simulink model "MEEN432_Project4_Model_V2"  (R2024b)
settings: Solver=VariableStepAuto  StartTime=0.0  StopTime=3600  RelTol=1e-3
values from neighbouring files (symbols this model uses):
  mph2mps = 1600/3600    (= 0.444444444444)    [Project4_init.m]
  x_track = zeros(size(s))    [Project4_track.m]
  y_track = zeros(size(s))    [Project4_track.m]
undefined symbols (not defined in the file or in its folder): datBat, datCar, datMotor
libraries: slpidlib x1
settings Model: Creator=flare  LastModifiedBy=jpalm
settings RTWCC: GPUComputeCapability=3.5

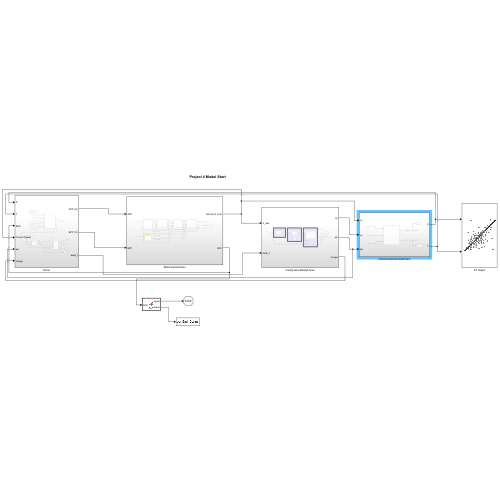
[thumbnail: Simulink's stored preview of the top-level diagram]
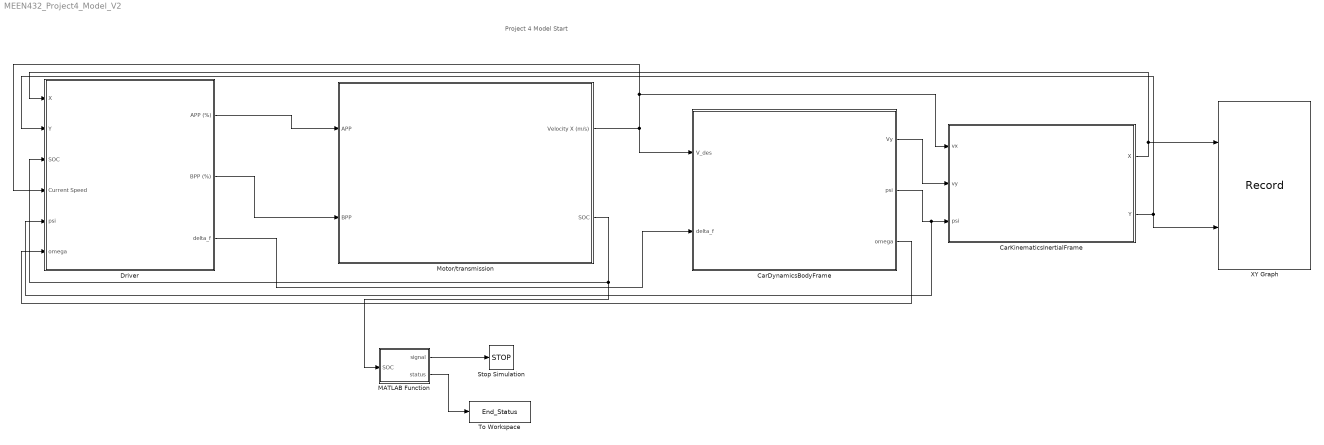
== system MEEN432_Project4_Model_V2 ==
  note: Project 4 Model Start
  CarDynamicsBodyFrame : Subsystem
  CarKinematicsInertialFrame : Subsystem
  Driver : Subsystem
  MATLAB Function : MATLAB Function  TreatAsAtomicUnit=on
  Motor/transmission : Subsystem
  Stop Simulation : Stop
  To Workspace : ToWorkspace  VariableName=End_Status  SaveFormat=Timeseries  SampleTime=-1
  XY Graph : Record  FileSettingsInternal="{\"entries\":[{\"content\":{\"excelSettings\":{\"content\":{},\"type\":\"Streamout.ExcelSettings\"}},\"type\":\"Streamout.FileSettingStorage\",\"uuid\":\"\"}],\"packageUris\":[\"http:\\/\\/schema.mathworks.com\\/mf0\\/streamout_blocks\\/R2020a\"],\"version\":\"1.0\"}"  Layout=[1 1]  SignalsInternal="{\"entries\":[{\"content\":{\"signals\":[{\"content\":{\"blockPath\":[],\"dimensions\":[1],\"domain\":\"\",\"lineColor\":\"#4dbeee\",\"plots\":[ 1 ],\"port\":1,\"sid\":[\"\"],\"signalID\":1,\"signalName\":\"CarKinematicsInertialFrame:1\"},\"type\":\"RecordBlkView.Signal\",\"uuid\":\"\"},{\"content\":{\"blockPath\":[],\"dimensions\":[1],\"domain\":\"\",\"lineColor\":\"#a2142f\",\"plots\":[ 1 ],\"port\":2,\"sid\":[\"\"],\"signalID\":2,\"signalName\":\"CarKinematicsInertialFrame:2\"},\"type\":\"RecordBlkView.Signal\",\"uuid\":\"\"}]},\"type\":\"RecordBlkView.InputSignals\",\"uuid\":\"\"}],\"packageUris\":[\"http:\\/\\/schema.mathworks.com\\/mf0\\/streamout_blocks\\/R2020a\"],\"version\":\"1.0\"}"  VisualizationBindings="{\"xyplotplugin\":{\"info\":[{\"series\":[{\"bindingParametersList\":[{\"parameter\":\"X-Axis\",\"signalID\":1,\"signalName\":\"CarKinematicsInertialFrame:1\"},{\"parameter\":\"Y-Axis\",\"signalID\":2,\"signalName\":\"CarKinematicsInertialFrame:2\"}],\"seriesID\":0}],\"subplotID\":1}]}}"  CompatibilityTag=XY
  wires:
  CarKinematicsInertialFrame/1(X) -> XY Graph/1, Driver/1(X)
  CarKinematicsInertialFrame/2(Y) -> XY Graph/2, Driver/2(Y)
  Driver/1(APP (%)) -> Motor/transmission/1(APP)
  Driver/2(BPP (%)) -> Motor/transmission/2(BPP)
  Driver/3(delta_f) -> CarDynamicsBodyFrame/2(delta_f)
  Motor/transmission/1(Velocity X (m/s)) -> Driver/4(Current Speed), CarKinematicsInertialFrame/1(vx), CarDynamicsBodyFrame/1(V_des)
  CarDynamicsBodyFrame/1(Vy) -> CarKinematicsInertialFrame/2(vy)
  CarDynamicsBodyFrame/2(psi) -> Driver/5(psi), CarKinematicsInertialFrame/3(psi)
  CarDynamicsBodyFrame/3(omega) -> Driver/6(omega)
  Motor/transmission/2(SOC) -> MATLAB Function/1(SOC), Driver/3(SOC)
  MATLAB Function/1(signal) -> Stop Simulation/1
  MATLAB Function/2(status) -> To Workspace/1

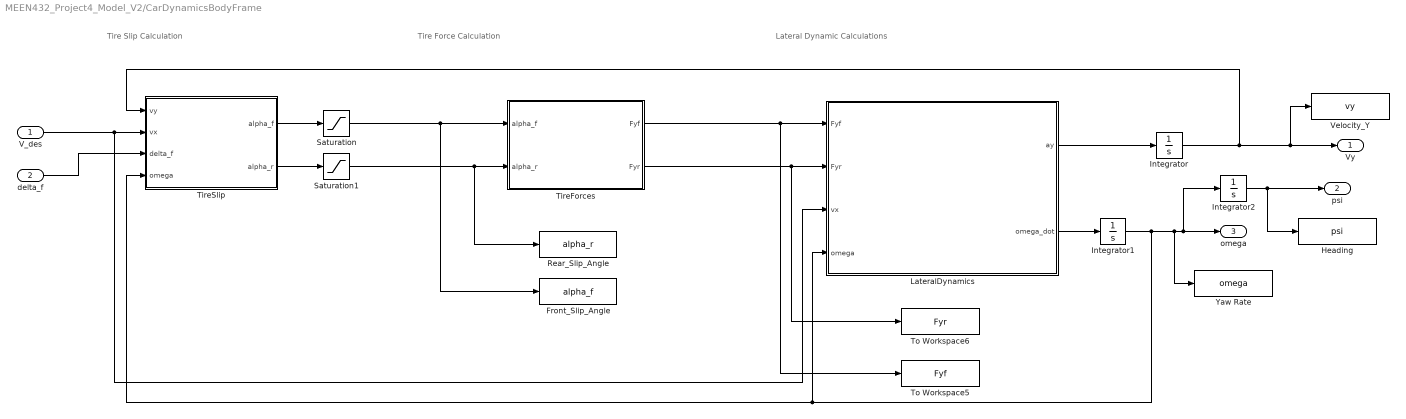
== system MEEN432_Project4_Model_V2/CarDynamicsBodyFrame ==
  note: Lateral Dynamic Calculations
  note: Tire Force Calculation
  note: Tire Slip Calculation
  V_des : Inport
  delta_f : Inport  Port=2
  Front_Slip_Angle : ToWorkspace  VariableName=alpha_f  SaveFormat=Timeseries  SampleTime=-1
  Heading : ToWorkspace  VariableName=psi  SaveFormat=Timeseries  SampleTime=-1
  Integrator : Integrator  InitialCondition=datCar.init.vy0
  Integrator1 : Integrator  InitialCondition=datCar.init.omega0
  Integrator2 : Integrator  InitialCondition=datCar.init.psi0
  LateralDynamics : MATLAB Function  TreatAsAtomicUnit=on  mask{obj=datCar}
      mask prompts: obj "obj structure"
  Rear_Slip_Angle : ToWorkspace  VariableName=alpha_r  SaveFormat=Timeseries  SampleTime=-1
  Saturation : Saturate  UpperLimit=datCar.maxAlpha  LowerLimit=-datCar.maxAlpha
  Saturation1 : Saturate  UpperLimit=datCar.maxAlpha  LowerLimit=-datCar.maxAlpha
  TireForces : MATLAB Function  TreatAsAtomicUnit=on  mask{obj=datCar}
      mask prompts: obj "obj structure"
  TireSlip : MATLAB Function  TreatAsAtomicUnit=on  mask{obj=datCar}
      mask prompts: obj "obj structure"
  To Workspace5 : ToWorkspace  VariableName=Fyf  SaveFormat=Timeseries  SampleTime=-1
  To Workspace6 : ToWorkspace  VariableName=Fyr  SaveFormat=Timeseries  SampleTime=-1
  Velocity_Y : ToWorkspace  VariableName=vy  SaveFormat=Timeseries  SampleTime=-1
  Yaw Rate : ToWorkspace  VariableName=omega  SaveFormat=Timeseries  SampleTime=-1
  Vy : Outport
  psi : Outport  Port=2
  omega : Outport  Port=3
  wires:
  delta_f/1 -> TireSlip/3(delta_f)
  V_des/1 -> TireSlip/2(vx), LateralDynamics/3(vx)
  Integrator2/1 -> Heading/1, psi/1
  Integrator1/1 -> Integrator2/1, omega/1, Yaw Rate/1, LateralDynamics/4(omega), TireSlip/4(omega)
  Saturation1/1 -> TireForces/2(alpha_r), Rear_Slip_Angle/1
  Saturation/1 -> TireForces/1(alpha_f), Front_Slip_Angle/1
  TireForces/1(Fyf) -> LateralDynamics/1(Fyf), To Workspace5/1
  LateralDynamics/1(ay) -> Integrator/1
  TireSlip/2(alpha_r) -> Saturation1/1
  TireSlip/1(alpha_f) -> Saturation/1
  TireForces/2(Fyr) -> LateralDynamics/2(Fyr), To Workspace6/1
  Integrator/1 -> Vy/1, Velocity_Y/1, TireSlip/1(vy)
  LateralDynamics/2(omega_dot) -> Integrator1/1

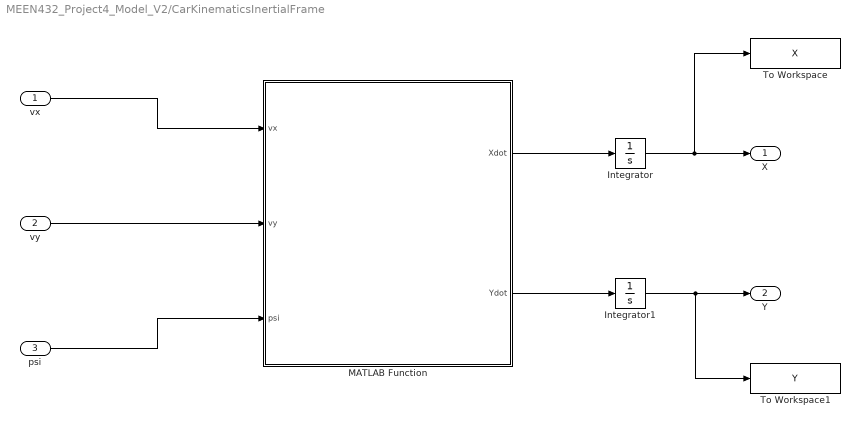
== system MEEN432_Project4_Model_V2/CarKinematicsInertialFrame ==
  vx : Inport
  vy : Inport  Port=2
  psi : Inport  Port=3
  Integrator : Integrator  InitialCondition=datCar.init.X0
  Integrator1 : Integrator  InitialCondition=datCar.init.Y0
  MATLAB Function : MATLAB Function  TreatAsAtomicUnit=on
  To Workspace : ToWorkspace  VariableName=X  SaveFormat=Timeseries  SampleTime=-1
  To Workspace1 : ToWorkspace  VariableName=Y  SaveFormat=Timeseries  SampleTime=-1
  X : Outport
  Y : Outport  Port=2
  wires:
  MATLAB Function/2(Ydot) -> Integrator1/1
  psi/1 -> MATLAB Function/3(psi)
  vx/1 -> MATLAB Function/1(vx)
  Integrator/1 -> To Workspace/1, X/1
  MATLAB Function/1(Xdot) -> Integrator/1
  Integrator1/1 -> To Workspace1/1, Y/1
  vy/1 -> MATLAB Function/2(vy)

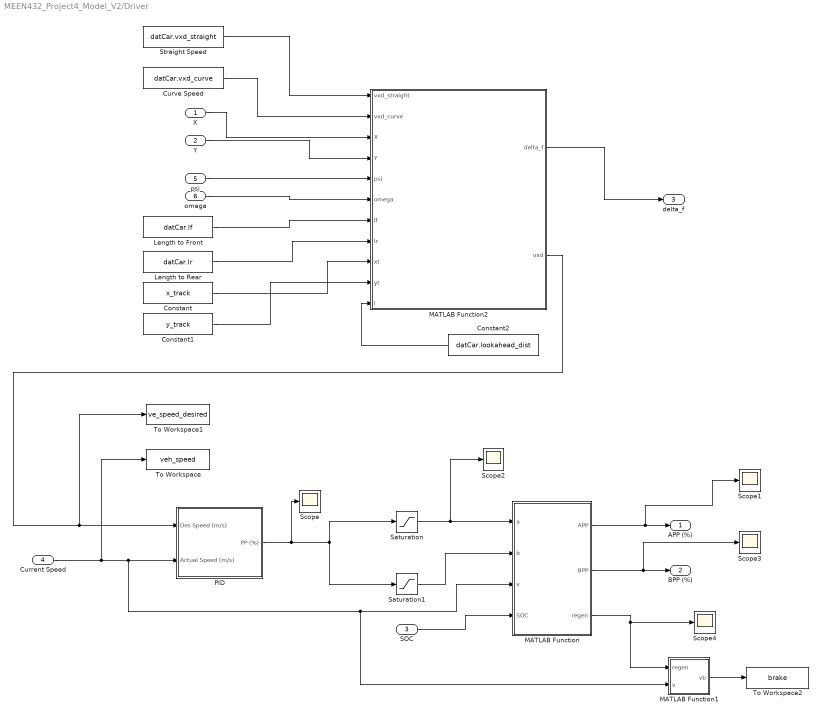
== system MEEN432_Project4_Model_V2/Driver ==
  X : Inport
  Y : Inport  Port=2
  SOC : Inport  Port=3
  Current Speed : Inport  Port=4
  psi : Inport  Port=5
  omega : Inport  Port=6
  Constant : Constant  Value=x_track  VectorParams1D=off
  Constant1 : Constant  Value=y_track  VectorParams1D=off
  Constant2 : Constant  Value=datCar.lookahead_dist
  Curve Speed : Constant  Value=datCar.vxd_curve
  Length to Front : Constant  Value=datCar.lf
  Length to Rear : Constant  Value=datCar.lr
  MATLAB Function : MATLAB Function  TreatAsAtomicUnit=on
  MATLAB Function1 : MATLAB Function  TreatAsAtomicUnit=on
  MATLAB Function2 : MATLAB Function  TreatAsAtomicUnit=on
  PID : Subsystem
  Saturation : Saturate  UpperLimit=1  LowerLimit=0
  Saturation1 : Saturate  UpperLimit=0  LowerLimit=-1
  Scope{,1..4} (5 alike) : Scope
  Straight Speed : Constant  Value=datCar.vxd_straight
  To Workspace : ToWorkspace  VariableName=veh_speed  SaveFormat=Timeseries  SampleTime=-1
  To Workspace1 : ToWorkspace  VariableName=ve_speed_desired  SaveFormat=Timeseries  SampleTime=-1
  To Workspace2 : ToWorkspace  VariableName=brake  SaveFormat=Timeseries  SampleTime=-1
  APP (%) : Outport
  BPP (%) : Outport  Port=2
  delta_f : Outport  Port=3
  wires:
  Current Speed/1 -> To Workspace/1, MATLAB Function1/2(v), MATLAB Function/3(v), PID/2(Actual Speed (m/s))
  MATLAB Function/1(APP) -> APP (%)/1, Scope1/1
  SOC/1 -> MATLAB Function/4(SOC)
  Saturation/1 -> Scope2/1, MATLAB Function/1(a)
  MATLAB Function/3(regen) -> MATLAB Function1/1(regen), Scope4/1
  MATLAB Function/2(BPP) -> BPP (%)/1, Scope3/1
  Saturation1/1 -> MATLAB Function/2(b)
  PID/1(PP (%)) -> Scope/1, Saturation1/1, Saturation/1
  MATLAB Function1/1(vb) -> To Workspace2/1
  Constant2/1 -> MATLAB Function2/11(l)
  Constant/1 -> MATLAB Function2/9(xt)
  Length to Rear/1 -> MATLAB Function2/8(lr)
  MATLAB Function2/1(delta_f) -> delta_f/1
  Constant1/1 -> MATLAB Function2/10(yt)
  X/1 -> MATLAB Function2/3(X)
  Y/1 -> MATLAB Function2/4(Y)
  Length to Front/1 -> MATLAB Function2/7(lf)
  Straight Speed/1 -> MATLAB Function2/1(vxd_straight)
  omega/1 -> MATLAB Function2/6(omega)
  psi/1 -> MATLAB Function2/5(psi)
  MATLAB Function2/2(vxd) -> To Workspace1/1, PID/1(Des Speed (m/s))
  Curve Speed/1 -> MATLAB Function2/2(vxd_curve)

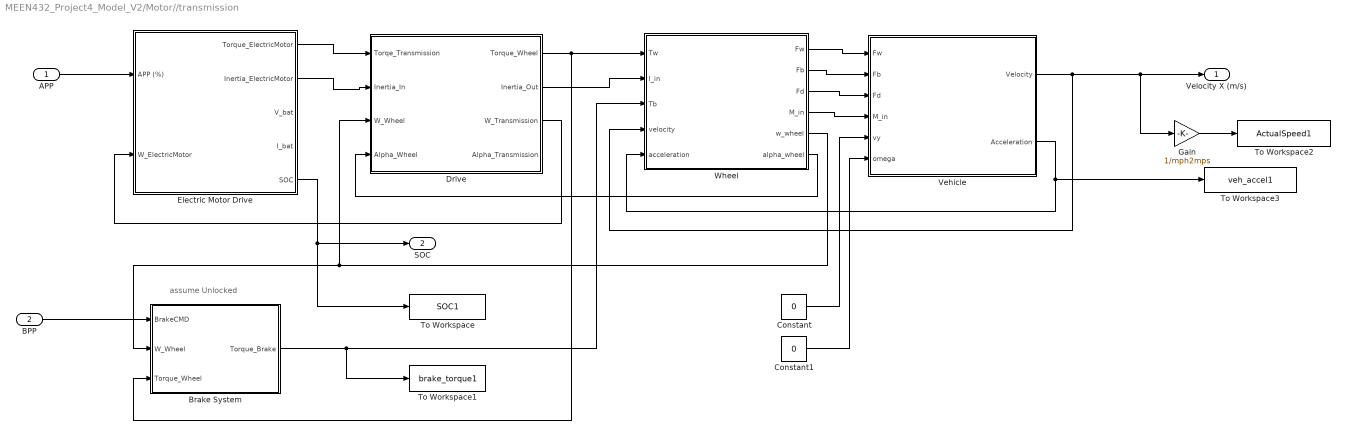
== system MEEN432_Project4_Model_V2/Motor//transmission ==
  note: assume Unlocked
  APP : Inport
  BPP : Inport  Port=2
  Brake System : Subsystem
  Constant : Constant  Value=0
  Constant1 : Constant  Value=0
  Drive : Subsystem
  Electric Motor Drive : Subsystem
  Gain : Gain  Gain=1/mph2mps
  To Workspace : ToWorkspace  VariableName=SOC1  SaveFormat=Timeseries  SampleTime=-1
  To Workspace1 : ToWorkspace  VariableName=brake_torque1  SaveFormat=Timeseries  SampleTime=-1
  To Workspace2 : ToWorkspace  VariableName=ActualSpeed1  SaveFormat=Timeseries  SampleTime=-1
  To Workspace3 : ToWorkspace  VariableName=veh_accel1  SaveFormat=Timeseries  SampleTime=-1
  Vehicle : Subsystem
  Wheel : Subsystem
  Velocity X (m/s) : Outport
  SOC : Outport  Port=2
  wires:
  Drive/3(W_Transmission) -> Electric Motor Drive/2(W_ElectricMotor)
  Drive/1(Torque_Wheel) -> Brake System/3(Torque_Wheel), Wheel/1(Tw)
  Brake System/1(Torque_Brake) -> To Workspace1/1, Wheel/3(Tb)
  Drive/2(Inertia_Out) -> Wheel/2(I_in)
  Wheel/1(Fw) -> Vehicle/1(Fw)
  Wheel/3(Fd) -> Vehicle/3(Fd)
  APP/1 -> Electric Motor Drive/1(APP (%))
  Vehicle/1(Velocity) -> Wheel/4(velocity), Gain/1, Velocity X (m/s)/1
  Wheel/2(Fb) -> Vehicle/2(Fb)
  Constant/1 -> Vehicle/5(vy)
  BPP/1 -> Brake System/1(BrakeCMD)
  Vehicle/2(Acceleration) -> To Workspace3/1, Wheel/5(acceleration)
  Electric Motor Drive/2(Inertia_ElectricMotor) -> Drive/2(Inertia_In)
  Gain/1 -> To Workspace2/1
  Constant1/1 -> Vehicle/6(omega)
  Electric Motor Drive/1(Torque_ElectricMotor) -> Drive/1(Torqe_Transmission)
  Wheel/6(alpha_wheel) -> Drive/4(Alpha_Wheel)
  Wheel/4(M_in) -> Vehicle/4(M_in)
  Electric Motor Drive/5(SOC) -> To Workspace/1, SOC/1
  Wheel/5(w_wheel) -> Drive/3(W_Wheel), Brake System/2(W_Wheel)

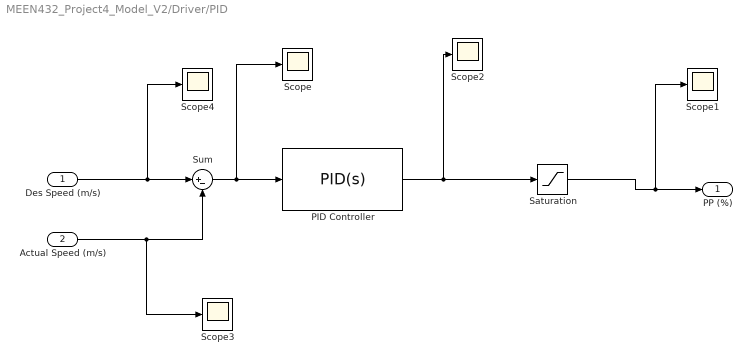
== system MEEN432_Project4_Model_V2/Driver/PID ==
  Des Speed (m/s) : Inport
  Actual Speed (m/s) : Inport  Port=2
  PID Controller : slpidlib/PID Controller  Controller=PID  Form=Parallel  TimeDomain=Continuous-time  UseExternalTs=off  SampleTime=-1  IntegratorMethod=Forward Euler  FilterMethod=Forward Euler  ControllerParametersSource=internal  P=1  I=1  UseKiTs=off  D=0  UseExternalDerivativeSource=off  N=100  UseFilter=on  TunerSelectOption=Transfer Function Based (PID Tuner App)  InitialConditionSource=internal  InitialConditionForIntegrator=0  InitialConditionForFilter=0  DifferentiatorICPrevScaledInput=0  ExternalReset=none  TrackingMode=off  Kt=1  LimitOutput=off  SatLimitsSource=internal  UpperSaturationLimit=inf  LowerSaturationLimit=-inf  LinearizeAsGain=on  AntiWindupMode=none  Kb=1  LimitIntegrator=off  UpperIntegratorSaturationLimit=inf  LowerIntegratorSaturationLimit=-inf  POutMin=[]  POutMax=[]  IOutMin=[]  IOutMax=[]  DOutMin=[]  DOutMax=[]  NOutMin=[]  NOutMax=[]  SumOutMin=[]  SumOutMax=[]  SaturationOutMin=[]  SaturationOutMax=[]  PParamMin=[]  PParamMax=[]  IParamMin=[]  IParamMax=[]  DParamMin=[]  DParamMax=[]  NParamMin=[]  NParamMax=[]  KbParamMin=[]  KbParamMax=[]  KtParamMin=[]  KtParamMax=[]  KbOutMin=[]  KbOutMax=[]  KtOutMin=[]  KtOutMax=[]  IntegratorOutMin=[]  IntegratorOutMax=[]  FilterOutMin=[]  FilterOutMax=[]  SumI1OutMin=[]  SumI1OutMax=[]  SumI2OutMin=[]  SumI2OutMax=[]  SumI3OutMin=[]  SumI3OutMax=[]  SumI4OutMin=[]  SumI4OutMax=[]  SumDOutMin=[]  SumDOutMax=[]  DifferentiatorOutMin=[]  DifferentiatorOutMax=[]  FilterDiffOutCoefMin=[]  FilterDiffOutCoefMax=[]  ReciprocalOutMin=[]  ReciprocalOutMax=[]  SumDenOutMin=[]  SumDenOutMax=[]  SumNumOutMin=[]  SumNumOutMax=[]  DivideOutMin=[]  DivideOutMax=[]  UdiffTsProdOutMin=[]  UdiffTsProdOutMax=[]  NTsProdOutMin=[]  NTsProdOutMax=[]  UintegralTsProdOutMin=[]  UintegralTsProdOutMax=[]  UngainTsProdOutMin=[]  UngainTsProdOutMax=[]  ClampingZeroOutDataTypeStr=Inherit: Inherit via back propagation  ClampingZeroOutMin=[]  ClampingZeroOutMax=[]  FilterDenConstantOutDataTypeStr=Inherit: Inherit via back propagation  FilterDenConstantOutMin=[]  FilterDenConstantOutMax=[]  PCopyOutDataTypeStr=Inherit: Inherit via back propagation  PCopyOutMin=[]  PCopyOutMax=[]  NCopyOutDataTypeStr=Inherit: Inherit via back propagation  NCopyOutMin=[]  NCopyOutMax=[]  IntegratorContinuousStateAttributes=''  IntegratorStateMustResolveToSignalObject=off  IntegratorRTWStateStorageClass=Auto  FilterContinuousStateAttributes=''  FilterStateMustResolveToSignalObject=off  FilterRTWStateStorageClass=Auto  ParallelPVariant=InternalParameters  IdealPVariant=Disabled  IVariant=InternalParameters  DVariant=InternalParameters  IntegratorVariant=Continuous  SatVariant=Disabled  AWVariant=Passthrough  PCopyVariant=Disabled  TRVariant=Disabled  FdbkBlocksVariant=Forward  IdealPFdbkVariant=Disabled  SatFdbkVariant=Disabled  DerivativeFilterVariant=ContFilter  NVariant=InternalParameters  NCopyVariant=Disabled  FilterICVariant=InternalICsFilter  IntegratorICVariant=InternalICs  ExternalResetVariant=Disabled  TRSumVariant=Passthrough  SumFdbkVariant=Disabled  SumVariant=Sum_PID  TsampFilterVariant=InternalTs  TsampNgainVariant=Passthrough  TsampIntegralVariant=Disabled_SignalSpec  ExternalSaturationOutDataTypeStr=Inherit: Same as second input  DerivativeSourceVariant=ErrorSignal  PreIntVariant=InternalPreInt
  Saturation : Saturate  UpperLimit=1  LowerLimit=-1
  Scope{,1..4} (5 alike) : Scope
  Sum : Sum  Inputs=|+-
  PP (%) : Outport
  wires:
  Sum/1 -> Scope/1, PID Controller/1
  PID Controller/1 -> Saturation/1, Scope2/1
  Des Speed (m/s)/1 -> Scope4/1, Sum/1
  Actual Speed (m/s)/1 -> Scope3/1, Sum/2
  Saturation/1 -> Scope1/1, PP (%)/1

== system MEEN432_Project4_Model_V2/Motor//transmission/Brake System ==
  BrakeCMD : Inport
  W_Wheel : Inport  Port=2
  Torque_Wheel : Inport  Port=3
  Constant : Constant  Value=datCar.maxBrakeTorque
  Constant1 : Constant  Value=datCar.brakeGeometricDesign
  Constant2 : Constant  Value=datCar.brakeFriction
  MATLAB Function : MATLAB Function  TreatAsAtomicUnit=on
  Scope : Scope
  Torque_Brake : Outport
  wires:
  BrakeCMD/1 -> MATLAB Function/1(alpha_b)
  W_Wheel/1 -> MATLAB Function/5(omega_w)
  MATLAB Function/1(tau_b) -> Scope/1, Torque_Brake/1
  Constant/1 -> MATLAB Function/3(N_b_max)
  Constant1/1 -> MATLAB Function/4(g_b)
  Constant2/1 -> MATLAB Function/2(mu_b)

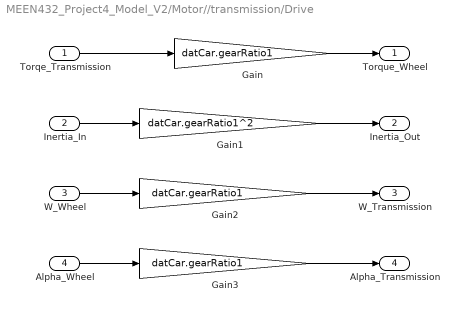
== system MEEN432_Project4_Model_V2/Motor//transmission/Drive ==
  Torqe_Transmission : Inport
  Inertia_In : Inport  Port=2
  W_Wheel : Inport  Port=3
  Alpha_Wheel : Inport  Port=4
  Gain : Gain  Gain=datCar.gearRatio1
  Gain1 : Gain  Gain=datCar.gearRatio1^2
  Gain2 : Gain  Gain=datCar.gearRatio1
  Gain3 : Gain  Gain=datCar.gearRatio1
  Torque_Wheel : Outport
  Inertia_Out : Outport  Port=2
  W_Transmission : Outport  Port=3
  Alpha_Transmission : Outport  Port=4
  wires:
  Torqe_Transmission/1 -> Gain/1
  Inertia_In/1 -> Gain1/1
  W_Wheel/1 -> Gain2/1
  Alpha_Wheel/1 -> Gain3/1
  Gain3/1 -> Alpha_Transmission/1
  Gain2/1 -> W_Transmission/1
  Gain1/1 -> Inertia_Out/1
  Gain/1 -> Torque_Wheel/1

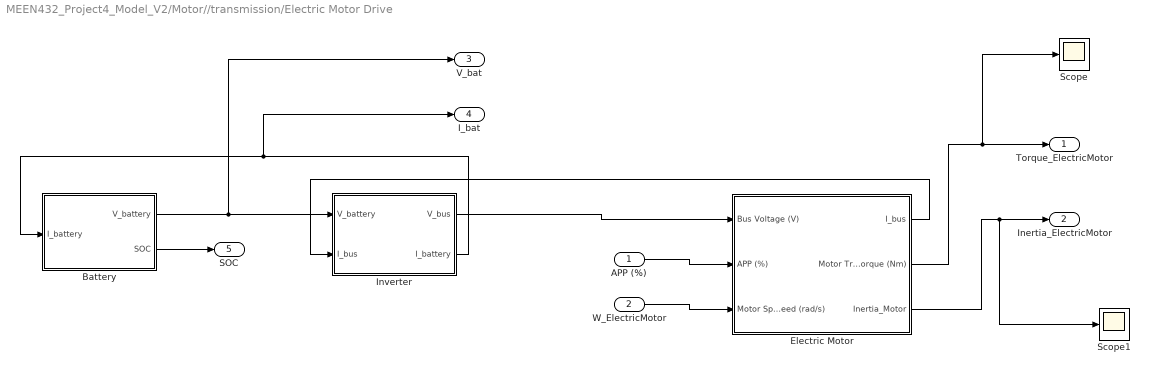
== system MEEN432_Project4_Model_V2/Motor//transmission/Electric Motor Drive ==
  APP (%) : Inport
  W_ElectricMotor : Inport  Port=2
  Battery : Subsystem
  Electric Motor : Subsystem
  Inverter : Subsystem
  Scope : Scope
  Scope1 : Scope
  Torque_ElectricMotor : Outport
  Inertia_ElectricMotor : Outport  Port=2
  V_bat : Outport  Port=3
  I_bat : Outport  Port=4
  SOC : Outport  Port=5
  wires:
  APP (%)/1 -> Electric Motor/2(APP (%))
  W_ElectricMotor/1 -> Electric Motor/3(Motor Speed (rad/s))
  Inverter/1(V_bus) -> Electric Motor/1(Bus Voltage (V))
  Battery/1(V_battery) -> V_bat/1, Inverter/1(V_battery)
  Inverter/2(I_battery) -> I_bat/1, Battery/1(I_battery)
  Electric Motor/1(I_bus) -> Inverter/2(I_bus)
  Electric Motor/2(Motor Trorque (Nm)) -> Scope/1, Torque_ElectricMotor/1
  Electric Motor/3(Inertia_Motor) -> Scope1/1, Inertia_ElectricMotor/1
  Battery/2(SOC) -> SOC/1

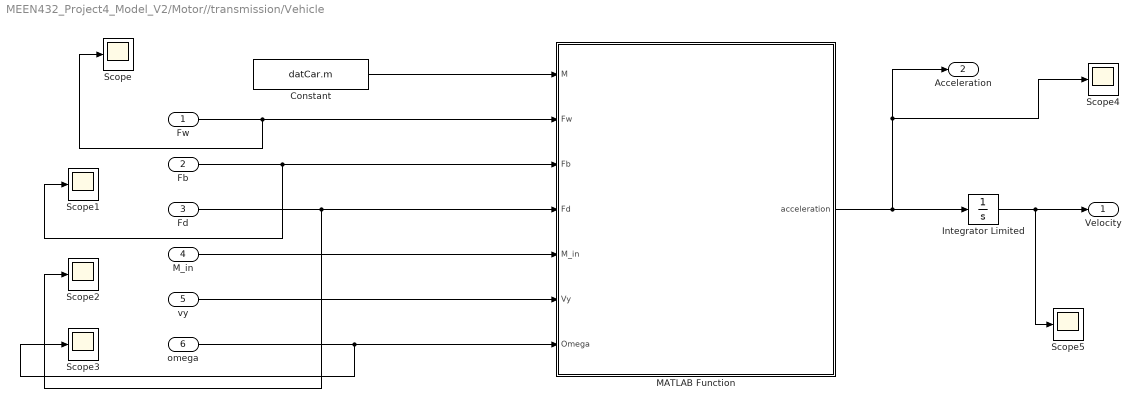
== system MEEN432_Project4_Model_V2/Motor//transmission/Vehicle ==
  Fw : Inport
  Fb : Inport  Port=2
  Fd : Inport  Port=3
  M_in : Inport  Port=4
  vy : Inport  Port=5
  omega : Inport  Port=6
  Constant : Constant  Value=datCar.m
  Integrator Limited : Integrator  LimitOutput=on  UpperSaturationLimit=10000  LowerSaturationLimit=0
  MATLAB Function : MATLAB Function  TreatAsAtomicUnit=on
  Scope{,1..5} (6 alike) : Scope
  Velocity : Outport
  Acceleration : Outport  Port=2
  wires:
  omega/1 -> Scope3/1, MATLAB Function/7(Omega)
  vy/1 -> MATLAB Function/6(Vy)
  M_in/1 -> MATLAB Function/5(M_in)
  Fb/1 -> Scope1/1, MATLAB Function/3(Fb)
  Fw/1 -> Scope/1, MATLAB Function/2(Fw)
  MATLAB Function/1(acceleration) -> Integrator Limited/1, Scope4/1, Acceleration/1
  Integrator Limited/1 -> Scope5/1, Velocity/1
  Constant/1 -> MATLAB Function/1(M)
  Fd/1 -> Scope2/1, MATLAB Function/4(Fd)

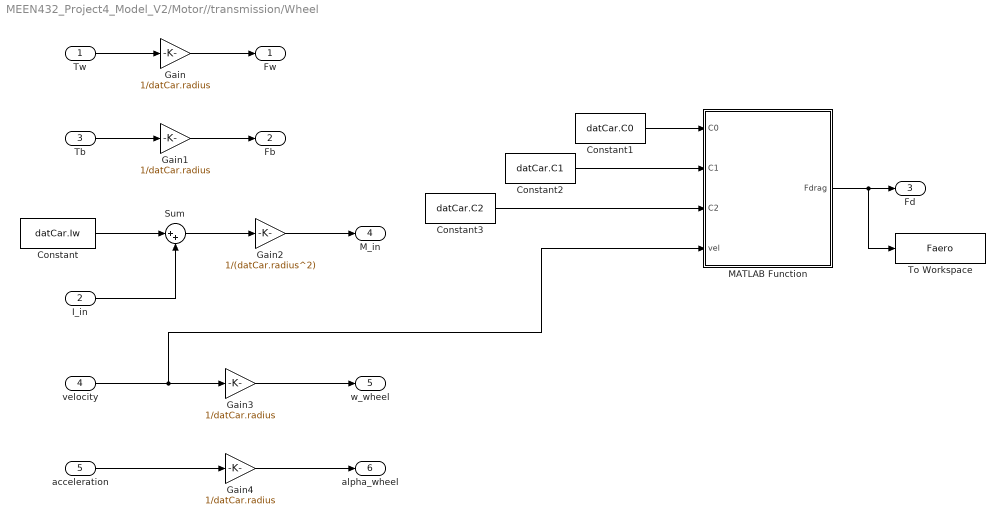
== system MEEN432_Project4_Model_V2/Motor//transmission/Wheel ==
  Tw : Inport
  I_in : Inport  Port=2
  Tb : Inport  Port=3
  velocity : Inport  Port=4
  acceleration : Inport  Port=5
  Constant : Constant  Value=datCar.Iw
  Constant1 : Constant  Value=datCar.C0
  Constant2 : Constant  Value=datCar.C1
  Constant3 : Constant  Value=datCar.C2
  Gain{,1,3..4} (4 alike) : Gain  Gain=1/datCar.radius
  Gain2 : Gain  Gain=1/(datCar.radius^2)
  MATLAB Function : MATLAB Function  TreatAsAtomicUnit=on
  Sum : Sum  Inputs=|++
  To Workspace : ToWorkspace  VariableName=Faero  SaveFormat=Timeseries  SampleTime=-1
  Fw : Outport
  Fb : Outport  Port=2
  Fd : Outport  Port=3
  M_in : Outport  Port=4
  w_wheel : Outport  Port=5
  alpha_wheel : Outport  Port=6
  wires:
  Tw/1 -> Gain/1
  Gain/1 -> Fw/1
  Gain1/1 -> Fb/1
  Tb/1 -> Gain1/1
  Constant/1 -> Sum/1
  I_in/1 -> Sum/2
  Sum/1 -> Gain2/1
  Gain2/1 -> M_in/1
  velocity/1 -> MATLAB Function/4(vel), Gain3/1
  acceleration/1 -> Gain4/1
  Gain3/1 -> w_wheel/1
  Gain4/1 -> alpha_wheel/1
  MATLAB Function/1(Fdrag) -> To Workspace/1, Fd/1
  Constant1/1 -> MATLAB Function/1(C0)
  Constant2/1 -> MATLAB Function/2(C1)
  Constant3/1 -> MATLAB Function/3(C2)

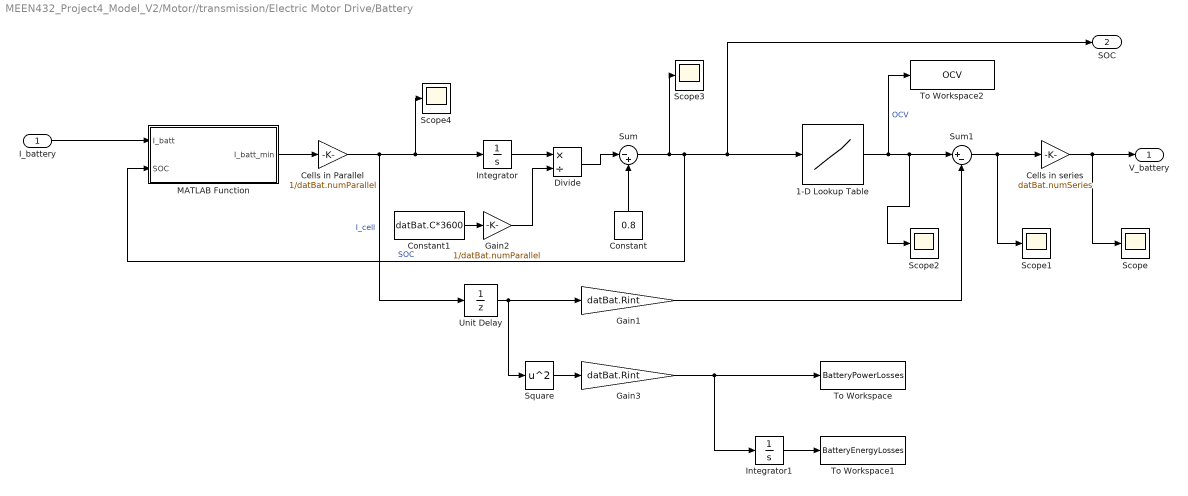
== system MEEN432_Project4_Model_V2/Motor//transmission/Electric Motor Drive/Battery ==
  I_battery : Inport
  1-D Lookup Table : Lookup_n-D  NumberOfTableDimensions=1  BreakpointsForDimension1=datBat.SOC  Table=datBat.OCV  InternalRulePriority=Speed  RndMeth=Simplest
  Cells in Parallel : Gain  Gain=1/datBat.numParallel
  Cells in series : Gain  Gain=datBat.numSeries
  Constant : Constant  Value=0.8
  Constant1 : Constant  Value=datBat.C*3600
  Divide : Product  Inputs=*/
  Gain1 : Gain  Gain=datBat.Rint
  Gain2 : Gain  Gain=1/datBat.numParallel
  Gain3 : Gain  Gain=datBat.Rint
  Integrator : Integrator
  Integrator1 : Integrator
  MATLAB Function : MATLAB Function  TreatAsAtomicUnit=on
  Scope{,1..4} (5 alike) : Scope
  Square : Math  Operator=square
  Sum : Sum  Inputs=|-+
  Sum1 : Sum  Inputs=|+-
  To Workspace : ToWorkspace  VariableName=BatteryPowerLosses  SaveFormat=Timeseries  SampleTime=-1
  To Workspace1 : ToWorkspace  VariableName=BatteryEnergyLosses  SaveFormat=Timeseries  SampleTime=-1
  To Workspace2 : ToWorkspace  VariableName=OCV  SaveFormat=Timeseries  SampleTime=-1
  Unit Delay : UnitDelay  SampleTime=-1  HasFrameUpgradeWarning=on
  V_battery : Outport
  SOC : Outport  Port=2
  wires:
  I_battery/1 -> MATLAB Function/1(I_batt)
  Cells in Parallel/1 -> Scope4/1, Integrator/1, Unit Delay/1  "I_cell"
  Unit Delay/1 -> Square/1, Gain1/1
  Constant/1 -> Sum/2
  Sum/1 -> Scope3/1, MATLAB Function/2(SOC), SOC/1, 1-D Lookup Table/1  "SOC"
  Constant1/1 -> Gain2/1
  Gain3/1 -> Integrator1/1, To Workspace/1
  Integrator1/1 -> To Workspace1/1
  Square/1 -> Gain3/1
  1-D Lookup Table/1 -> To Workspace2/1, Scope2/1, Sum1/1  "OCV"
  Gain1/1 -> Sum1/2
  Sum1/1 -> Scope1/1, Cells in series/1
  Cells in series/1 -> Scope/1, V_battery/1
  Integrator/1 -> Divide/1
  Gain2/1 -> Divide/2
  Divide/1 -> Sum/1
  MATLAB Function/1(I_batt_min) -> Cells in Parallel/1

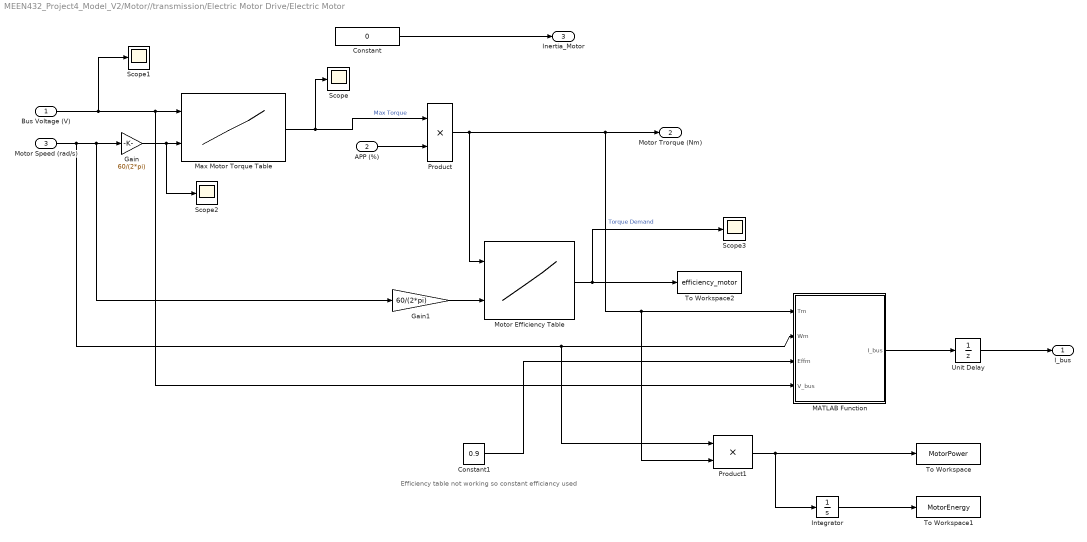
== system MEEN432_Project4_Model_V2/Motor//transmission/Electric Motor Drive/Electric Motor ==
  note: Efficiency table not working so constant efficiancy used
  Bus Voltage (V) : Inport
  APP (%) : Inport  Port=2
  Motor Speed (rad/s) : Inport  Port=3
  Constant : Constant  Value=0
  Constant1 : Constant  Value=0.9
  Gain : Gain  Gain=60/(2*pi)
  Gain1 : Gain  Gain=60/(2*pi)
  Integrator : Integrator
  MATLAB Function : MATLAB Function  TreatAsAtomicUnit=on
  Max Motor Torque Table : Lookup_n-D  BreakpointsForDimension1=datMotor.vbus  BreakpointsForDimension2=datMotor.rpm  Table=datMotor.maxtorque  InternalRulePriority=Speed  RndMeth=Simplest
      settings: InputPortMap=u0,u1
  Motor Efficiency Table : Lookup_n-D  BreakpointsForDimension1=datMotor.eta_torque  BreakpointsForDimension2=datMotor.eta_speed  Table=datMotor.eta_val  InternalRulePriority=Speed  RndMeth=Simplest
      settings: InputPortMap=u0,u1
  Product : Product
  Product1 : Product
  Scope{,1..3} (4 alike) : Scope
  To Workspace : ToWorkspace  VariableName=MotorPower  SaveFormat=Timeseries  SampleTime=-1
  To Workspace1 : ToWorkspace  VariableName=MotorEnergy  SaveFormat=Timeseries  SampleTime=-1
  To Workspace2 : ToWorkspace  VariableName=efficiency_motor  SaveFormat=Timeseries  SampleTime=-1
  Unit Delay : UnitDelay  SampleTime=-1  HasFrameUpgradeWarning=on
  I_bus : Outport
  Motor Trorque (Nm) : Outport  Port=2
  Inertia_Motor : Outport  Port=3
  wires:
  Bus Voltage (V)/1 -> Scope1/1, MATLAB Function/4(V_bus), Max Motor Torque Table/1
  Motor Speed (rad/s)/1 -> Gain/1, Gain1/1, Product1/1, MATLAB Function/2(Wm)
  Gain/1 -> Scope2/1, Max Motor Torque Table/2
  Max Motor Torque Table/1 -> Scope/1, Product/1  "Max Torque"
  APP (%)/1 -> Product/2
  Constant/1 -> Inertia_Motor/1
  Product/1 -> Product1/2, MATLAB Function/1(Tm), Motor Trorque (Nm)/1, Motor Efficiency Table/1  "Torque Demand"
  Gain1/1 -> Motor Efficiency Table/2
  Motor Efficiency Table/1 -> Scope3/1, To Workspace2/1
  Unit Delay/1 -> I_bus/1
  MATLAB Function/1(I_bus) -> Unit Delay/1
  Product1/1 -> Integrator/1, To Workspace/1
  Integrator/1 -> To Workspace1/1
  Constant1/1 -> MATLAB Function/3(Effm)

== system MEEN432_Project4_Model_V2/Motor//transmission/Electric Motor Drive/Inverter ==
  V_battery : Inport
  I_bus : Inport  Port=2
  Efficiency Inverter : Constant  Value=0.95
  MATLAB Function : MATLAB Function  TreatAsAtomicUnit=on
  Scope : Scope
  Scope1 : Scope
  V_bus : Outport
  I_battery : Outport  Port=2
  wires:
  V_battery/1 -> Scope1/1, MATLAB Function/1(V_bat)
  Efficiency Inverter/1 -> MATLAB Function/2(Eff_I)
  I_bus/1 -> MATLAB Function/3(I_bus)
  MATLAB Function/1(V_bus) -> Scope/1, V_bus/1
  MATLAB Function/2(I_bat) -> I_battery/1

== matlab function MEEN432_Project4_Model_V2/Driver/MATLAB Function ==
  data: a input; APP output; b input; v input; SOC input; BPP output; regen output
function [APP, BPP, regen] = fcn(a, b, v, SOC)
    if v < (5*(1600/3600))
        regen = 0;
        APP = 1;
        BPP = -b;
    elseif v == (25*(1600/3600))
        regen = 0.95;
        friction = 0.05;
        APP = 1 + b*regen;
        BPP = -b*friction;
    elseif v > (25*(1600/3600))
        regen = 0.95;
        friction = 0.05;
        APP = a + b*regen;
        BPP = -b*friction;
    else regen = (0.95/20)*v;
        friction = 1 - regen;
        APP = a + b*regen;
        BPP = -b*friction;
    end

    if SOC <= 0.1
        APP = 0;
        BPP = 0;
        regen = 0;
    end

== matlab function MEEN432_Project4_Model_V2/Driver/MATLAB Function1 ==
  data: regen input; vb output; v input
function vb = fcn(regen, v)

vb = regen*v;

== matlab function MEEN432_Project4_Model_V2/Motor//transmission/Electric Motor Drive/Electric Motor/MATLAB Function ==
  data: Tm input; I_bus output; Wm input; Effm input; V_bus input
function I_bus = fcn(Tm, Wm, Effm, V_bus)
    Pm = Tm*Wm;
    sgn_m = Pm / (abs(Pm) + 0.001);
    Pe = Pm / (Effm^sgn_m);
    if V_bus > 1
        I_bus = Pe/V_bus;
    else
        I_bus = 0;
    end

== matlab function MEEN432_Project4_Model_V2/Motor//transmission/Electric Motor Drive/Inverter/MATLAB Function ==
  data: V_bat input; V_bus output; Eff_I input; I_bus input; I_bat output
function [V_bus, I_bat] = fcn(V_bat, Eff_I, I_bus)
    V_bus = V_bat; % Vbus = Vbat * r, where r is the inverter conversion ratio % * I_bat * Eff_I^(sgn_Pbat))/I_bus;
    P_bus = V_bus * I_bus;
    sgn_Pbus = P_bus / (abs(P_bus) + 0.001);

    if V_bus > 1
        I_bat = (P_bus / Eff_I^sgn_Pbus) / V_bat;
    else
        I_bat = 0;
    end
end

% double check ?

== matlab function MEEN432_Project4_Model_V2/Motor//transmission/Vehicle/MATLAB Function ==
  data: M input; acceleration output; Fw input; Fb input; Fd input; M_in input; Vy input; Omega input
function acceleration = fcn(M, Fw, Fb, Fd, M_in, Vy, Omega)

acceleration = ((Fw - Fb - Fd) / (M + M_in)) + Vy*Omega;

== matlab function MEEN432_Project4_Model_V2/Motor//transmission/Wheel/MATLAB Function ==
  data: C0 input; Fdrag output; C1 input; C2 input; vel input
function Fdrag = fcn(C0, C1, C2, vel)

Fdrag = C0 + C1*vel + C2*vel^2;

== matlab function MEEN432_Project4_Model_V2/CarDynamicsBodyFrame/TireForces ==
  data: alpha_f input; alpha_r input; Fyf output; obj parameter; Fyr output
function [Fyf, Fyr] = fcn(alpha_f, alpha_r, obj)

Fyf = min(obj.Fyfmax,obj.Calpha_f * alpha_f);
Fyr = min(obj.Fyrmax, obj.Calpha_r * alpha_r);
end

== matlab function MEEN432_Project4_Model_V2/Driver/MATLAB Function2 ==
  data: vxd_straight input; vxd_curve input; X input; delta_f output; Y input; psi input; omega input; lf input; lr input; xt input; yt input; l input; vxd output
function [delta_f, vxd]= fcn(vxd_straight, vxd_curve, X, Y, psi, omega, lf, lr, xt, yt, l)

    % Initialize parameters
    car_loc = [X, Y];
    track = [xt; yt];
    base = lf + lr;
    
    % Find closest track point
    dist = vecnorm(track - car_loc');
    [~, closest] = min(dist);
    
    % Set look-ahead window
    look_ahead = l;
    curve_window = 15;  % Points to analyze for curve detection
    threshold = 2.5;    % Meters of Y variation to trigger curve
    
    % Get upcoming track segment
    start_idx = closest;
    end_idx = min(closest + look_ahead + curve_window, length(track));
    y_segment = track(2, start_idx:end_idx);
    
    % Detect curve using Y variation
    y_variation = max(y_segment) - min(y_segment);
    is_curve = y_variation > threshold;
    
    % Select appropriate speed
    vxd = vxd_curve * is_curve + vxd_straight * ~is_curve;
    
    % Calculate target point
    target_idx = min(closest + look_ahead, length(track));
    target = track(:, target_idx);
    
    % Calculate steering angle
    alpha = atan2(target(2)-Y, target(1)-X) - psi;
    psi_dot = 2*vxd*sin(alpha)/base;
    delta_f = psi_dot - omega;
end

== matlab function MEEN432_Project4_Model_V2/CarDynamicsBodyFrame/TireSlip ==
  data: vy input size=1; vx input; delta_f input size=1; omega input; alpha_f output; obj parameter; alpha_r output
function [alpha_f, alpha_r] = fcn(vy,  vx, delta_f, omega, obj)

if abs(vx)> obj.vx_threshold1
      alpha_f = delta_f - (vy + omega * obj.lf) / vx;
      alpha_r = - (vy - omega * obj.lr) / vx;
else
      alpha_f = 0;
      alpha_r = 0;
end
end
% if abs(vx)> obj.vx_threshold1
%       alpha_f = delta_f - atan2(vy + omega * obj.lf,vx);
%       alpha_r = atan2(vy - omega * obj.lr,vx);
% else
%       alpha_f = 0;
%       alpha_r = 0;
% end
% end

== matlab function MEEN432_Project4_Model_V2/Motor//transmission/Brake System/MATLAB Function ==
  data: alpha_b input; tau_b output; mu_b input; N_b_max input; g_b input; omega_w input
function tau_b = fcn(alpha_b, mu_b, N_b_max, g_b, omega_w)

N_b = alpha_b * N_b_max;
sgn = omega_w/(omega_w+0.0001);
tau_b = mu_b * N_b * g_b * sgn;

== matlab function MEEN432_Project4_Model_V2/CarKinematicsInertialFrame/MATLAB Function ==
  data: vx input; Xdot output; vy input; psi input; Ydot output
function [Xdot, Ydot] = fcn(vx, vy, psi)

%velocity matrix
v = [vx; vy];
%rotation matrix
rot = [cos(psi), -sin(psi); sin(psi), cos(psi)];

temp = rot * v;

%rotated velocity matrix
Xdot = temp(1);
Ydot = temp(2);

== matlab function MEEN432_Project4_Model_V2/CarDynamicsBodyFrame/LateralDynamics ==
  data: Fyf input; Fyr input size=1; vx input; omega input; ay output; obj parameter; omega_dot output
function [ay, omega_dot] = fcn(Fyf, Fyr, vx, omega, obj)

Fy = Fyf + Fyr;
ay = Fy / obj.m - omega * vx;
        
M  = Fyf * obj.lf - Fyr * obj.lr;        
omega_dot = M / obj.I;        

end

== matlab function MEEN432_Project4_Model_V2/Motor//transmission/Electric Motor Drive/Battery/MATLAB Function ==
  data: I_batt input; I_batt_min output; SOC input
function I_batt_min = fcn(I_batt, SOC)
    if SOC <= 0.1
        I_batt_min = 0;
    else
        I_batt_min = I_batt;
    end

== matlab function MEEN432_Project4_Model_V2/MATLAB Function ==
  data: SOC input; signal output; status output
function [signal, status]= fcn(SOC)

signal = 0;
status = 0;

if SOC <= 0.1
    status = 1;
    signal = 1;
end
